simulink model "fourier_example"  (R2013b)
settings: Solver=FixedStepDiscrete  StartTime=0.0  StopTime=0.1  FixedStep=1/100000  MaxStep=10/1000  RelTol=1e-3
undefined symbols (not defined in the file or in its folder): Fs, get
libraries: dspspect3 x1, dspsnks4 x1
settings Model: Creator=eg572583  LastModifiedBy=ChrisJobling
settings DataIOCC: SignalLoggingSaveFormat=ModelDataLogs
settings DebuggingCC: MultiTaskDSMMsg=warning  MultiTaskCondExecSysMsg=none
settings RTWCC: IncludeERTFirstTime=on

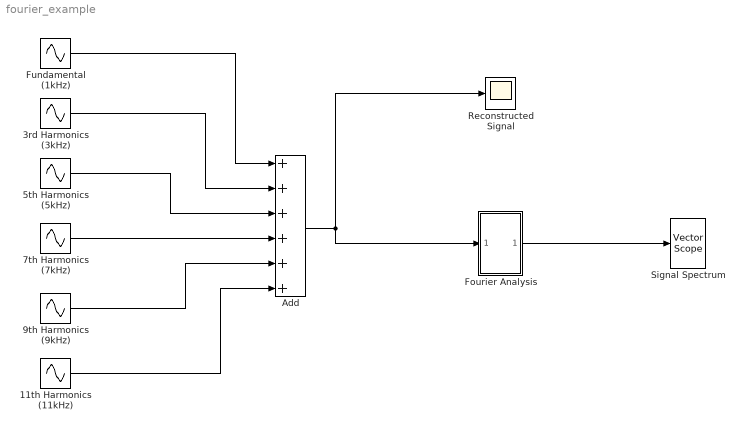
== system fourier_example ==
  11th Harmonics (11kHz) : Sin  Amplitude=0.1157  Frequency=11000*2*pi  SampleTime=0
  3rd Harmonics (3kHz) : Sin  Amplitude=0.4244  Frequency=3*1000*2*pi  SampleTime=0
  5th Harmonics (5kHz) : Sin  Amplitude=0.2546  Frequency=5000*2*pi  SampleTime=0
  7th Harmonics (7kHz) : Sin  Amplitude=0.1819  Frequency=7000*2*pi  SampleTime=0
  9th Harmonics (9kHz) : Sin  Amplitude=0.1415  Frequency=9000*2*pi  SampleTime=0
  Add : Sum  Inputs=++++++
  Fourier Analysis : Subsystem
  Fundamental (1kHz) : Sin  Amplitude=1.273  Frequency=1000*2*pi  SampleTime=0
  Reconstructed Signal : Scope
      settings: YMin=-2  YMax=2
  Signal Spectrum : dspsnks4/Vector Scope  ScopeProperties=on  Domain=Frequency  HorizSpan=1  DisplayProperties=off  AxisGrid=on  Memory=off  FrameNumber=on  AxisLegend=off  AxisZoom=off  OpenScopeAtSimStart=on  OpenScopeImmediately=off  FigPos=get(0,'defaultfigureposition')  AxisProperties=off  XUnits=Hertz  XRange=[-Fs/2...Fs/2]  InheritXIncr=on  XIncr=1  XLabel=Time  XLimit=Auto  XMin=0  XMax=4  XStart=0  YUnits=Magnitude  YLabel=Amplitude  LineProperties=off  LineMarkers=o  XAxisParamsVer=6.9
      settings: YMin=0  YMax=20
  wires:
  Fundamental (1kHz)/1 -> Add/1
  3rd Harmonics (3kHz)/1 -> Add/2
  5th Harmonics (5kHz)/1 -> Add/3
  7th Harmonics (7kHz)/1 -> Add/4
  9th Harmonics (9kHz)/1 -> Add/5
  11th Harmonics (11kHz)/1 -> Add/6
  Add/1 -> Fourier Analysis/1(In1), Reconstructed Signal/1
  Fourier Analysis/1(Out1) -> Signal Spectrum/1

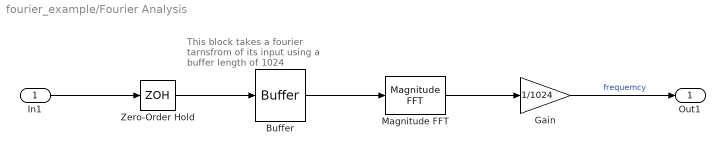
== system fourier_example/Fourier Analysis ==
  note: This block takes a fourier tarnsfrom of its input using a buffer length of 1024
  In1 : Inport
  Buffer : Buffer  N=1024  TreatMby1Signals=One channel
  Gain : Gain  Gain=1/1024
  Magnitude FFT : dspspect3/Magnitude FFT  mag_or_magsq=Magnitude  FFTImplementation=Auto  fftLenInherit=off  fftsize=1024
  Zero-Order Hold : ZeroOrderHold  SampleTime=50e-6
  Out1 : Outport
  wires:
  Magnitude FFT/1 -> Gain/1
  Gain/1 -> Out1/1  "frequemcy"
  In1/1 -> Zero-Order Hold/1
  Zero-Order Hold/1 -> Buffer/1
  Buffer/1 -> Magnitude FFT/1
